simulink model "Simulate"  (R2024b)
settings: Solver=VariableStepAuto  StartTime=0.0  StopTime=Tf  FixedStep=Ti  MaxStep=Ti  RelTol=1e-6
undefined symbols (not defined in the file): CCMPC, CEMPC, DiscIntNeverNeededParam, dspblkCoreblockFVToolHelper, FOC, gcbh, IM, KF, LPF, M2C, plecs, PLL, RFT, TEB, Ti, Ts
libraries: slpidlib x4, spsdq0toAlphaBetaZeroLib x3, dspstat3 x2, spsAlphaBetaZerotoabcLib x2, embmathops x1, spsabctodq0Lib x1, spsAlphaBetaZerotodq0Lib x1, spsabctoAlphaBetaZeroLib x1
(part 1 of 2)
settings Model: Creator=Pablo  LastModifiedBy=Ingeniería Eléctrica
settings SolverCC: MinimalZcImpactIntegration=on

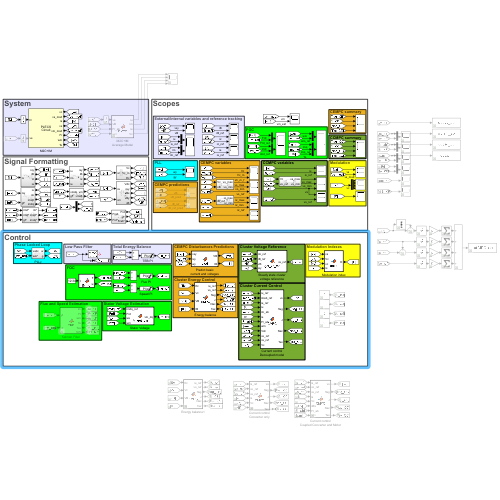
[thumbnail: Simulink's stored preview of the top-level diagram]
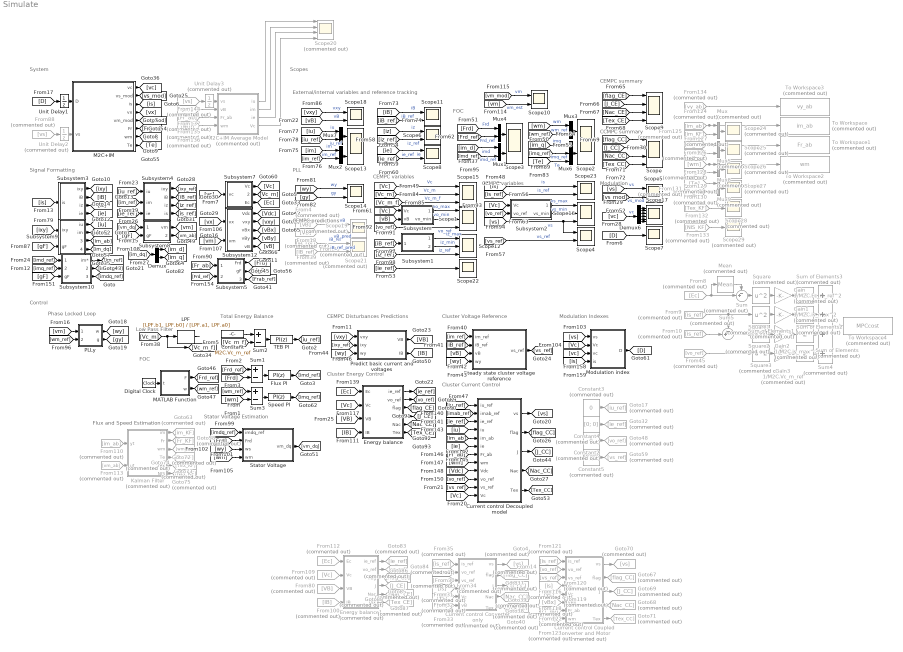
== system Simulate ==
  note: Control
  note: System
  note: Signal Formatting
  note: Scopes
  note: CEMPC predictions
  note: CEMPC variables
  note: External/internal variables and reference tracking
  note: CEMPC Disturbances Predictions
  note: FOC
  note: Cluster Energy Control
  note: Cluster Current Control
  note: Phase Locked Loop
  note: Low Pass Filter
  note: Cluster Voltage Reference
  note: PLL
  note: CEMPC summary
  note: CCMPC summary
  note: Total Energy Balance
  note: FOC
  note: CCMPC variables
  note: Modulation Indexes
  note: Flux and Speed Estimation
  note: Stator Voltage Estimation
  note: Modulation
  Constant : Constant  Value=M2C.Vc_m_ref  SampleTime=TEB.Ts
  Constant2 : Constant  Commented=on  Value=0  SampleTime=Ts
  Constant3 : Constant  Commented=on  Value=0  SampleTime=Ts
  Constant4 : Constant  Commented=on  Value=[0; 0]  SampleTime=Ts
  Constant5 : Constant  Commented=on  Value=zeros(6, 1)  SampleTime=Ts
  Current control Converter only : MATLAB Function  Commented=on  TreatAsAtomicUnit=on  SystemSampleTime=CCMPC.Ts
  Current control Coupled Converter and Motor : MATLAB Function  Commented=on  TreatAsAtomicUnit=on  SystemSampleTime=CCMPC.Ts
  Current control Decoupled model : MATLAB Function  TreatAsAtomicUnit=on  SystemSampleTime=CCMPC.Ts
  Demux : Demux  Outputs=2
  Demux6 : Demux  Outputs=M2C.m
  Digital Clock : DigitalClock  SampleTime=FOC.Ts
  Energy balance : MATLAB Function  TreatAsAtomicUnit=on  SystemSampleTime=CEMPC.Ts
  Energy balance1 : MATLAB Function  Commented=on  TreatAsAtomicUnit=on  SystemSampleTime=CEMPC.Ts
  Flux PI : slpidlib/PID Controller  Controller=PI  Form=Parallel  TimeDomain=Discrete-time  UseExternalTs=off  SampleTime=FOC.Ts  IntegratorMethod=Forward Euler  FilterMethod=Forward Euler  ControllerParametersSource=internal  P=FOC.kp_F  I=FOC.ki_F  UseKiTs=off  D=0  UseExternalDerivativeSource=off  N=100  UseFilter=on  TunerSelectOption=Transfer Function Based (PID Tuner App)  InitialConditionSource=internal  InitialConditionForIntegrator=0  InitialConditionForFilter=0  DifferentiatorICPrevScaledInput=0  ExternalReset=none  TrackingMode=off  Kt=1  LimitOutput=on  SatLimitsSource=internal  UpperSaturationLimit=FOC.u_max  LowerSaturationLimit=FOC.u_min  LinearizeAsGain=on  AntiWindupMode=back-calculation  Kb=FOC.kp_F  LimitIntegrator=off  UpperIntegratorSaturationLimit=inf  LowerIntegratorSaturationLimit=-inf  POutMin=[]  POutMax=[]  IOutMin=[]  IOutMax=[]  DOutMin=[]  DOutMax=[]  NOutMin=[]  NOutMax=[]  SumOutMin=[]  SumOutMax=[]  SaturationOutMin=[]  SaturationOutMax=[]  PParamMin=[]  PParamMax=[]  IParamMin=[]  IParamMax=[]  DParamMin=[]  DParamMax=[]  NParamMin=[]  NParamMax=[]  KbParamMin=[]  KbParamMax=[]  KtParamMin=[]  KtParamMax=[]  KbOutMin=[]  KbOutMax=[]  KtOutMin=[]  KtOutMax=[]  IntegratorOutMin=[]  IntegratorOutMax=[]  FilterOutMin=[]  FilterOutMax=[]  SumI1OutMin=[]  SumI1OutMax=[]  SumI2OutMin=[]  SumI2OutMax=[]  SumI3OutMin=[]  SumI3OutMax=[]  SumI4OutMin=[]  SumI4OutMax=[]  SumDOutMin=[]  SumDOutMax=[]  DifferentiatorOutMin=[]  DifferentiatorOutMax=[]  FilterDiffOutCoefMin=[]  FilterDiffOutCoefMax=[]  ReciprocalOutMin=[]  ReciprocalOutMax=[]  SumDenOutMin=[]  SumDenOutMax=[]  SumNumOutMin=[]  SumNumOutMax=[]  DivideOutMin=[]  DivideOutMax=[]  UdiffTsProdOutMin=[]  UdiffTsProdOutMax=[]  NTsProdOutMin=[]  NTsProdOutMax=[]  UintegralTsProdOutMin=[]  UintegralTsProdOutMax=[]  UngainTsProdOutMin=[]  UngainTsProdOutMax=[]  ClampingZeroOutDataTypeStr=Inherit: Inherit via back propagation  ClampingZeroOutMin=[]  ClampingZeroOutMax=[]  FilterDenConstantOutDataTypeStr=Inherit: Inherit via back propagation  FilterDenConstantOutMin=[]  FilterDenConstantOutMax=[]  PCopyOutDataTypeStr=Inherit: Inherit via back propagation  PCopyOutMin=[]  PCopyOutMax=[]  NCopyOutDataTypeStr=Inherit: Inherit via back propagation  NCopyOutMin=[]  NCopyOutMax=[]  IntegratorContinuousStateAttributes=''  IntegratorStateMustResolveToSignalObject=off  IntegratorRTWStateStorageClass=Auto  FilterContinuousStateAttributes=''  FilterStateMustResolveToSignalObject=off  FilterRTWStateStorageClass=Auto  ParallelPVariant=InternalParameters  IdealPVariant=Disabled  IVariant=InternalParameters  DVariant=Disabled  IntegratorVariant=Discrete  SatVariant=Enabled  AWVariant=BackCalculation  PCopyVariant=Disabled  TRVariant=Disabled  FdbkBlocksVariant=Forward  IdealPFdbkVariant=Disabled  SatFdbkVariant=Disabled  DerivativeFilterVariant=Disabled  NVariant=Disabled  NCopyVariant=Disabled_SignalSpec  FilterICVariant=Disabled  IntegratorICVariant=InternalICs  ExternalResetVariant=Disabled  TRSumVariant=Passthrough  SumFdbkVariant=Disabled  SumVariant=Sum_PI  TsampFilterVariant=InternalTs  TsampNgainVariant=Passthrough  TsampIntegralVariant=Disabled_SignalSpec  ExternalSaturationOutDataTypeStr=Inherit: Same as second input  DerivativeSourceVariant=Disabled  PreIntVariant=InternalPreInt
  From{9..10,35,121} (4 alike) : From  Commented=on  GotoTag=is_ref
  From100 : From  Commented=on  GotoTag=IB
  From109 : From  Commented=on  GotoTag=Vc
  From110 : From  Commented=on  GotoTag=im_ab
  From112 : From  Commented=on  GotoTag=Ec
  From113 : From  Commented=on  GotoTag=vm_ab
  From116 : From  Commented=on  GotoTag=vs_ref
  From118 : From  Commented=on  GotoTag=Vc
  From119 : From  Commented=on  GotoTag=vBx
  From120 : From  Commented=on  GotoTag=is
  From122 : From  Commented=on  GotoTag=Fr_ab
  From123 : From  Commented=on  GotoTag=wm
  From124 : From  Commented=on  GotoTag=im_ab
  From125 : From  Commented=on  GotoTag=im_KF
  From126 : From  Commented=on  GotoTag=Fr_ab
  From127 : From  Commented=on  GotoTag=Fr_KF
  From128 : From  Commented=on  GotoTag=wm
  From129 : From  Commented=on  GotoTag=wm_KF
  From130 : From  Commented=on  GotoTag=Te
  From131 : From  Commented=on  GotoTag=Te_KF
  From132 : From  Commented=on  GotoTag=Tex_KF
  From133 : From  Commented=on  GotoTag=NIS_KF
  From134 : From  Commented=on  GotoTag=vy_ab
  From135 : From  Commented=on  GotoTag=Fr_ab
  From136 : From  Commented=on  GotoTag=wm
  From137 : From  Commented=on  GotoTag=vB
  From14 : From  Commented=on  GotoTag=vo_ref
  From144 : From  Commented=on  GotoTag=vs
  From18 : From  Commented=on  GotoTag=VB
  From30 : From  Commented=on  GotoTag=vo_ref
  From31 : From  Commented=on  GotoTag=vs_ref
  From32 : From  Commented=on  GotoTag=Vc
  From33 : From  Commented=on  GotoTag=vB
  From34 : From  Commented=on  GotoTag=is
  From36 : From  Commented=on  GotoTag=IB_ref
  From39 : From  Commented=on  GotoTag=iB_ref
  From4 : From  Commented=on  GotoTag=vB
  From45 : From  Commented=on  GotoTag=vo_ref
  From8 : From  Commented=on  GotoTag=Ec
  From80 : From  Commented=on  GotoTag=VB
  From88 : From  Commented=on  GotoTag=vs
  Gain : Gain  Commented=on  Gain=1/M2C.Ec_m_ref^2
  Gain1 : Gain  Commented=on  Gain=1/M2C.is_max^2
  Gain2 : Gain  Commented=on  Gain=1/M2C.is_max^2
  Gain3 : Gain  Commented=on  Gain=1/M2C.Vc_m_ref
  Goto17 : Goto  Commented=on  GotoTag=iu_ref
  Goto32 : Goto  Commented=on  GotoTag=ie_ref
  Goto37 : Goto  Commented=on  GotoTag=flag_CC
  Goto38 : Goto  Commented=on  GotoTag=Nac_CC
  Goto39 : Goto  Commented=on  GotoTag=J_CC
  Goto4 : Goto  Commented=on  GotoTag=vs
  Goto40 : Goto  Commented=on  GotoTag=Tex_CC
  Goto48 : Goto  Commented=on  GotoTag=vo_ref
  Goto58 : Goto  Commented=on  GotoTag=Fr_KF
  Goto59 : Goto  Commented=on  GotoTag=vs_ref
  Goto63 : Goto  Commented=on  GotoTag=im_KF
  Goto67 : Goto  Commented=on  GotoTag=flag_CC
  Goto68 : Goto  Commented=on  GotoTag=Nac_CC
  Goto69 : Goto  Commented=on  GotoTag=J_CC
  Goto70 : Goto  Commented=on  GotoTag=vs
  Goto71 : Goto  Commented=on  GotoTag=Tex_CC
  Goto72 : Goto  Commented=on  GotoTag=wm_KF
  Goto73 : Goto  Commented=on  GotoTag=Te_KF
  Goto74 : Goto  Commented=on  GotoTag=Tex_KF
  Goto75 : Goto  Commented=on  GotoTag=NIS_KF
  Goto83 : Goto  Commented=on  GotoTag=ie_ref
  Goto84 : Goto  Commented=on  GotoTag=vo_ref
  Goto85 : Goto  Commented=on  GotoTag=flag_CE
  Goto86 : Goto  Commented=on  GotoTag=J_CE
  Goto87 : Goto  Commented=on  GotoTag=Nac_CE
  Goto88 : Goto  Commented=on  GotoTag=Tex_CE
  Kalman Filter : MATLAB Function  Commented=on  TreatAsAtomicUnit=on  SystemSampleTime=FOC.Ts
  LPF : DiscreteTransferFcn  LoadFcn=dspblkCoreblockFVToolHelper(gcbh,'load');  Numerator=[LPF.b1, LPF.b0]  Denominator=[LPF.a1, LPF.a0]  InitialStates=M2C.Vc_m_ref*9.3230807
      settings: CopyFcn=dspblkCoreblockFVToolHelper(gcbh,'copy');  DeleteFcn=dspblkCoreblockFVToolHelper(gcbh,'close');  ModelCloseFcn=dspblkCoreblockFVToolHelper(gcbh,'close');  PreSaveFcn=dspblkCoreblockFVToolHelper(gcbh,'presave');  PostSaveFcn=dspblkCoreblockFVToolHelper(gcbh,'postsave');  CloseFcn=dspblkCoreblockFVToolHelper(gcbh,'close');
  M2C+IM : Subsystem  LoadFcn=plecs('sl', 200);  InitFcn=plecs('sl', 214);  StartFcn=plecs('sl', 208);  StopFcn=plecs('sl', 209);  mask(PlecsCircuit){PLECSData=<binary blob, 34036 chars, not shown>}
      mask prompts: PLECSData "PLECS Data (Do not delete or modify!)"
      mask init:
      | % PLACE CUSTOM INITIALIZATIONS ABOVE
      | % DO NOT REMOVE
      | plecs('sl', 215);
      | % DO NOT REMOVE
      settings: CopyFcn=plecs('sl', 203);  DeleteFcn=plecs('sl', 205);  UndoDeleteFcn=plecs('sl', 206);  PreSaveFcn=plecs('sl', 211);  PostSaveFcn=plecs('sl', 201);  NameChangeFcn=plecs('sl', 210);  DestroyFcn=plecs('sl', 207);  PreCopyFcn=plecs('sl', 216);  OpenFcn=plecs('sl', 202);  ErrorFcn=plerrorfcn
      mask Help: eval('plecs(''help'', ''qthelp:///creatingacircuit.html'')')
      mask Display: disp('PLECS\nCircuit')
  M2C+IM Average Model : MATLAB Function  Commented=on  TreatAsAtomicUnit=on  SystemSampleTime=CCMPC.Ts
  MATLAB Function : MATLAB Function  TreatAsAtomicUnit=on  SystemSampleTime=FOC.Ts
  Mean : dspstat3/Mean  Commented=on  run=off  InputProcessing=Columns as channels (frame based)  reset_popup=None  directionMode=Entire input  dimension=1  roiEnable=off  roiType=Rectangles  roiPortion=Entire ROI  roiOutput=Individual statistics for each ROI  roiFlag=off  roundingMode=Floor  overflowMode=off  outputDataTypeStr=Inherit: Same as accumulator  outputMin=[]  outputMax=[]  outputLastDataTypeStr=Inherit: Same as accumulator
  Modulation index : MATLAB Function  TreatAsAtomicUnit=on  SystemSampleTime=CCMPC.Ts
  Mux : Mux  Commented=on  Inputs=[2; 2]
  Mux{1,3..4,7} (4 alike) : Mux  Inputs=2
  Mux2 : Mux  Inputs=[3; 3]
  Mux5 : Mux  Commented=on  Inputs=[2; 2]
  Mux6 : Mux  Inputs=3
  Mux8 : Mux  Commented=on  Inputs=2
  Mux9 : Mux  Commented=on  Inputs=2
  PLLy : Subsystem
  Predict basic current and voltages : MATLAB Function  TreatAsAtomicUnit=on  SystemSampleTime=CEMPC.Ts
  Scope : Scope  NumInputPorts=4
  Scope{1,12,15..16} (4 alike) : Scope  NumInputPorts=3
  Scope{2..6,8,10..11,13..14,18,23} (12 alike) : Scope  NumInputPorts=2
  Scope17 : Scope  NumInputPorts=6
  Scope19 : Scope  Commented=on  NumInputPorts=2
  Scope20 : Scope  Commented=on  NumInputPorts=4
  Scope21 : Scope  Commented=on  NumInputPorts=2
  Scope22 : Scope
  Scope{24..29} (6 alike) : Scope  Commented=on
  Scope7 : Scope
  Scope9 : Scope  NumInputPorts=4
  Speed PI : slpidlib/PID Controller  Controller=PI  Form=Parallel  TimeDomain=Discrete-time  UseExternalTs=off  SampleTime=FOC.Ts  IntegratorMethod=Forward Euler  FilterMethod=Forward Euler  ControllerParametersSource=internal  P=FOC.kp_w  I=FOC.ki_w  UseKiTs=off  D=0  UseExternalDerivativeSource=off  N=100  UseFilter=on  TunerSelectOption=Transfer Function Based (PID Tuner App)  InitialConditionSource=internal  InitialConditionForIntegrator=0  InitialConditionForFilter=0  DifferentiatorICPrevScaledInput=0  ExternalReset=none  TrackingMode=off  Kt=1  LimitOutput=on  SatLimitsSource=internal  UpperSaturationLimit=FOC.u_max  LowerSaturationLimit=FOC.u_min  LinearizeAsGain=on  AntiWindupMode=back-calculation  Kb=FOC.kp_w  LimitIntegrator=off  UpperIntegratorSaturationLimit=inf  LowerIntegratorSaturationLimit=-inf  POutMin=[]  POutMax=[]  IOutMin=[]  IOutMax=[]  DOutMin=[]  DOutMax=[]  NOutMin=[]  NOutMax=[]  SumOutMin=[]  SumOutMax=[]  SaturationOutMin=[]  SaturationOutMax=[]  PParamMin=[]  PParamMax=[]  IParamMin=[]  IParamMax=[]  DParamMin=[]  DParamMax=[]  NParamMin=[]  NParamMax=[]  KbParamMin=[]  KbParamMax=[]  KtParamMin=[]  KtParamMax=[]  KbOutMin=[]  KbOutMax=[]  KtOutMin=[]  KtOutMax=[]  IntegratorOutMin=[]  IntegratorOutMax=[]  FilterOutMin=[]  FilterOutMax=[]  SumI1OutMin=[]  SumI1OutMax=[]  SumI2OutMin=[]  SumI2OutMax=[]  SumI3OutMin=[]  SumI3OutMax=[]  SumI4OutMin=[]  SumI4OutMax=[]  SumDOutMin=[]  SumDOutMax=[]  DifferentiatorOutMin=[]  DifferentiatorOutMax=[]  FilterDiffOutCoefMin=[]  FilterDiffOutCoefMax=[]  ReciprocalOutMin=[]  ReciprocalOutMax=[]  SumDenOutMin=[]  SumDenOutMax=[]  SumNumOutMin=[]  SumNumOutMax=[]  DivideOutMin=[]  DivideOutMax=[]  UdiffTsProdOutMin=[]  UdiffTsProdOutMax=[]  NTsProdOutMin=[]  NTsProdOutMax=[]  UintegralTsProdOutMin=[]  UintegralTsProdOutMax=[]  UngainTsProdOutMin=[]  UngainTsProdOutMax=[]  ClampingZeroOutDataTypeStr=Inherit: Inherit via back propagation  ClampingZeroOutMin=[]  ClampingZeroOutMax=[]  FilterDenConstantOutDataTypeStr=Inherit: Inherit via back propagation  FilterDenConstantOutMin=[]  FilterDenConstantOutMax=[]  PCopyOutDataTypeStr=Inherit: Inherit via back propagation  PCopyOutMin=[]  PCopyOutMax=[]  NCopyOutDataTypeStr=Inherit: Inherit via back propagation  NCopyOutMin=[]  NCopyOutMax=[]  IntegratorContinuousStateAttributes=''  IntegratorStateMustResolveToSignalObject=off  IntegratorRTWStateStorageClass=Auto  FilterContinuousStateAttributes=''  FilterStateMustResolveToSignalObject=off  FilterRTWStateStorageClass=Auto  ParallelPVariant=InternalParameters  IdealPVariant=Disabled  IVariant=InternalParameters  DVariant=Disabled  IntegratorVariant=Discrete  SatVariant=Enabled  AWVariant=BackCalculation  PCopyVariant=Disabled  TRVariant=Disabled  FdbkBlocksVariant=Forward  IdealPFdbkVariant=Disabled  SatFdbkVariant=Disabled  DerivativeFilterVariant=Disabled  NVariant=Disabled  NCopyVariant=Disabled_SignalSpec  FilterICVariant=Disabled  IntegratorICVariant=InternalICs  ExternalResetVariant=Disabled  TRSumVariant=Passthrough  SumFdbkVariant=Disabled  SumVariant=Sum_PI  TsampFilterVariant=InternalTs  TsampNgainVariant=Passthrough  TsampIntegralVariant=Disabled_SignalSpec  ExternalSaturationOutDataTypeStr=Inherit: Same as second input  DerivativeSourceVariant=Disabled  PreIntVariant=InternalPreInt
  Square{,1..3} (4 alike) : Math  Commented=on  Operator=square
  Stator Voltage : MATLAB Function  TreatAsAtomicUnit=on  SystemSampleTime=CCMPC.Ts
  Steady state cluster voltage reference : MATLAB Function  TreatAsAtomicUnit=on  SystemSampleTime=CCMPC.Ts
  Subsystem : Subsystem
  Subsystem1 : Subsystem
  Subsystem10 : Subsystem
  Subsystem12 : Subsystem
  Subsystem2 : Subsystem
  Subsystem3 : Subsystem
  Subsystem4 : Subsystem
  Subsystem5 : Subsystem
  Subsystem7 : Subsystem
  Subsystem8 : Subsystem
  Subsystem9 : Subsystem
  Sum : Sum  Commented=on  Inputs=-+|
  Sum of Elements{,1..3} (4 alike) : Sum  Commented=on  Inputs=+
  Sum1 : Sum  Inputs=+-
  Sum2 : Sum  Inputs=+-
  Sum3 : Sum  Inputs=+-
  Sum4 : Sum  Commented=on  Inputs=++++
  Sum5 : Sum  Commented=on  Inputs=-+|
  TEB PI : slpidlib/PID Controller  Controller=PI  Form=Parallel  TimeDomain=Discrete-time  UseExternalTs=off  SampleTime=TEB.Ts  IntegratorMethod=Forward Euler  FilterMethod=Forward Euler  ControllerParametersSource=internal  P=TEB.kp  I=TEB.ki  UseKiTs=off  D=0  UseExternalDerivativeSource=off  N=100  UseFilter=on  TunerSelectOption=Transfer Function Based (PID Tuner App)  InitialConditionSource=internal  InitialConditionForIntegrator=0  InitialConditionForFilter=0  DifferentiatorICPrevScaledInput=0  ExternalReset=none  TrackingMode=off  Kt=1  LimitOutput=on  SatLimitsSource=internal  UpperSaturationLimit=TEB.u_max  LowerSaturationLimit=TEB.u_min  LinearizeAsGain=on  AntiWindupMode=clamping  Kb=1  LimitIntegrator=off  UpperIntegratorSaturationLimit=inf  LowerIntegratorSaturationLimit=-inf  POutMin=[]  POutMax=[]  IOutMin=[]  IOutMax=[]  DOutMin=[]  DOutMax=[]  NOutMin=[]  NOutMax=[]  SumOutMin=[]  SumOutMax=[]  SaturationOutMin=[]  SaturationOutMax=[]  PParamMin=[]  PParamMax=[]  IParamMin=[]  IParamMax=[]  DParamMin=[]  DParamMax=[]  NParamMin=[]  NParamMax=[]  KbParamMin=[]  KbParamMax=[]  KtParamMin=[]  KtParamMax=[]  KbOutMin=[]  KbOutMax=[]  KtOutMin=[]  KtOutMax=[]  IntegratorOutMin=[]  IntegratorOutMax=[]  FilterOutMin=[]  FilterOutMax=[]  SumI1OutMin=[]  SumI1OutMax=[]  SumI2OutMin=[]  SumI2OutMax=[]  SumI3OutMin=[]  SumI3OutMax=[]  SumI4OutMin=[]  SumI4OutMax=[]  SumDOutMin=[]  SumDOutMax=[]  DifferentiatorOutMin=[]  DifferentiatorOutMax=[]  FilterDiffOutCoefMin=[]  FilterDiffOutCoefMax=[]  ReciprocalOutMin=[]  ReciprocalOutMax=[]  SumDenOutMin=[]  SumDenOutMax=[]  SumNumOutMin=[]  SumNumOutMax=[]  DivideOutMin=[]  DivideOutMax=[]  UdiffTsProdOutMin=[]  UdiffTsProdOutMax=[]  NTsProdOutMin=[]  NTsProdOutMax=[]  UintegralTsProdOutMin=[]  UintegralTsProdOutMax=[]  UngainTsProdOutMin=[]  UngainTsProdOutMax=[]  ClampingZeroOutDataTypeStr=Inherit: Inherit via back propagation  ClampingZeroOutMin=[]  ClampingZeroOutMax=[]  FilterDenConstantOutDataTypeStr=Inherit: Inherit via back propagation  FilterDenConstantOutMin=[]  FilterDenConstantOutMax=[]  PCopyOutDataTypeStr=Inherit: Inherit via back propagation  PCopyOutMin=[]  PCopyOutMax=[]  NCopyOutDataTypeStr=Inherit: Inherit via back propagation  NCopyOutMin=[]  NCopyOutMax=[]  IntegratorContinuousStateAttributes=''  IntegratorStateMustResolveToSignalObject=off  IntegratorRTWStateStorageClass=Auto  FilterContinuousStateAttributes=''  FilterStateMustResolveToSignalObject=off  FilterRTWStateStorageClass=Auto  ParallelPVariant=InternalParameters  IdealPVariant=Disabled  IVariant=InternalParameters  DVariant=Disabled  IntegratorVariant=Discrete  SatVariant=Enabled  AWVariant=DiscClampingParallel  PCopyVariant=Disabled  TRVariant=Disabled  FdbkBlocksVariant=Forward  IdealPFdbkVariant=Disabled  SatFdbkVariant=Disabled  DerivativeFilterVariant=Disabled  NVariant=Disabled  NCopyVariant=Disabled_SignalSpec  FilterICVariant=Disabled  IntegratorICVariant=InternalICs  ExternalResetVariant=Disabled  TRSumVariant=Passthrough  SumFdbkVariant=Disabled  SumVariant=Sum_PI  TsampFilterVariant=InternalTs  TsampNgainVariant=Passthrough  TsampIntegralVariant=Disabled_SignalSpec  ExternalSaturationOutDataTypeStr=Inherit: Same as second input  DerivativeSourceVariant=Disabled  PreIntVariant=InternalPreInt
  To Workspace : ToWorkspace  Commented=on  VariableName=im_ab  SaveFormat=Timeseries  SampleTime=FOC.Ts
  To Workspace1 : ToWorkspace  Commented=on  VariableName=Fr_ab  SaveFormat=Timeseries  SampleTime=FOC.Ts
  To Workspace2 : ToWorkspace  Commented=on  VariableName=wm  SaveFormat=Timeseries  SampleTime=FOC.Ts
  To Workspace3 : ToWorkspace  Commented=on  VariableName=vy_ab  SaveFormat=Timeseries  SampleTime=FOC.Ts
  To Workspace4 : ToWorkspace  Commented=on  VariableName=MPCcost  SaveFormat=Timeseries  SampleTime=Ts
  Unit Delay1 : UnitDelay  InitialCondition=zeros(24, 1)  SampleTime=Ti  HasFrameUpgradeWarning=on
  Unit Delay2 : UnitDelay  Commented=on  InitialCondition=zeros(6, 1)  SampleTime=Ti  HasFrameUpgradeWarning=on
  Unit Delay3 : UnitDelay  Commented=on  InitialCondition=zeros(6, 1)  SampleTime=Ti  HasFrameUpgradeWarning=on
  wires:
  From14/1 -> Current control Coupled Converter and Motor/2(vo_ref)
  From120/1 -> Current control Coupled Converter and Motor/4(is)
  From119/1 -> Current control Coupled Converter and Motor/6(vBx)
  Current control Coupled Converter and Motor/3(J) -> Goto69/1
  Current control Coupled Converter and Motor/2(flag) -> Goto67/1
  From121/1 -> Current control Coupled Converter and Motor/1(is_ref)
  Current control Coupled Converter and Motor/1(vs) -> Goto70/1
  Current control Coupled Converter and Motor/5(Tex) -> Goto71/1
  Current control Coupled Converter and Motor/4(Nac) -> Goto68/1
  From118/1 -> Current control Coupled Converter and Motor/5(Vc)
  From116/1 -> Current control Coupled Converter and Motor/3(vs_ref)
  From122/1 -> Current control Coupled Converter and Motor/7(Fr_ab)
  From123/1 -> Current control Coupled Converter and Motor/8(wm)
  From125/1 -> Mux/2
  From132/1 -> Scope28/1
  From126/1 -> To Workspace1/1, Mux5/1
  From131/1 -> Mux9/2
  From129/1 -> Mux8/2
  From130/1 -> Mux9/1
  From128/1 -> To Workspace2/1, Mux8/1
  From127/1 -> Mux5/2
  Mux/1 -> Scope24/1
  Mux5/1 -> Scope25/1
  Mux8/1 -> Scope26/1
  Mux9/1 -> Scope27/1
  From133/1 -> Scope29/1
  From124/1 -> To Workspace/1, Mux/1
  From134/1 -> To Workspace3/1
  From8/1 -> Sum/2, Mean/1
  Sum/1 -> Square/1
  From9/1 -> Sum5/1, Square1/1
  Square1/1 -> Gain1/1
  Square/1 -> Gain/1
  Square2/1 -> Gain2/1
  Mean/1 -> Sum/1
  From45/1 -> Square3/1
  Sum4/1 -> To Workspace4/1
  Sum5/1 -> Square2/1
  From10/1 -> Sum5/2
  Square3/1 -> Gain3/1
  Gain/1 -> Sum of Elements3/1
  Gain1/1 -> Sum of Elements2/1
  Gain2/1 -> Sum of Elements1/1
  Gain3/1 -> Sum of Elements/1
  Sum of Elements/1 -> Sum4/4
  Sum of Elements1/1 -> Sum4/3
  Sum of Elements2/1 -> Sum4/2
  Sum of Elements3/1 -> Sum4/1
  [iu] -> Current control Decoupled model/4(iu)
  [ie_ref] -> Current control Decoupled model/3(ie_ref)
  [imab_ref] -> Current control Decoupled model/2(imab_ref)
  [iu_ref] -> Current control Decoupled model/1(iu_ref)
  [im_ab] -> Current control Decoupled model/5(im_ab)
  [ie] -> Current control Decoupled model/6(ie)
  [Fr_ab] -> Current control Decoupled model/7(Fr_ab)
  [wm] -> Current control Decoupled model/8(wm)
  [Vdc] -> Current control Decoupled model/9(Vdc)
  [vo_ref] -> Current control Decoupled model/10(vo_ref)
  Current control Decoupled model/1(vs) -> [vs]
  [Vc] -> Current control Decoupled model/12(Vc)
  Current control Decoupled model/2(flag) -> [flag_CC]
  Current control Decoupled model/3(J) -> [J_CC]
  Current control Decoupled model/4(Nac) -> [Nac_CC]
  Current control Decoupled model/5(Tex) -> [Tex_CC]
  [vs_ref] -> Current control Decoupled model/11(vs_ref)
  Energy balance1/3(flag) -> Goto85/1
  Energy balance1/6(Tex) -> Goto88/1
  Energy balance1/4(J) -> Goto86/1
  Energy balance1/1(ie_ref) -> Goto83/1
  From80/1 -> Energy balance1/3(VB)
  From109/1 -> Energy balance1/2(Vc)
  Energy balance1/5(Nac) -> Goto87/1
  From112/1 -> Energy balance1/1(Ec)
  Energy balance1/2(vo_ref) -> Goto84/1
  From100/1 -> Energy balance1/4(IB)
  From31/1 -> Current control Converter only/3(vs_ref)
  From34/1 -> Current control Converter only/4(is)
  Current control Converter only/4(Nac) -> Goto38/1
  From33/1 -> Current control Converter only/6(vB)
  Current control Converter only/3(J) -> Goto39/1
  From32/1 -> Current control Converter only/5(Vc)
  From30/1 -> Current control Converter only/2(vo_ref)
  From35/1 -> Current control Converter only/1(is_ref)
  Current control Converter only/2(flag) -> Goto37/1
  Current control Converter only/5(Tex) -> Goto40/1
  Current control Converter only/1(vs) -> Goto4/1
  [im_dq] -> Demux/1
  Demux/2 -> [im_q]
  [gF] -> Subsystem10/3(gF)
  [imq_ref] -> Subsystem10/2(imq*)
  Demux/1 -> [im_d]
  Subsystem10/1(im*) -> [im_ref]
  PLLy/1(w) -> [wy]
  Subsystem/2(vo_min) -> Scope1/2  "vo_min"
  [vs_mod] -> Scope5/2  "vs_mod"
  [wm_ref] -> PLLy/2(wm*)
  [ixy_ref] -> Predict basic current and voltages/2(ixy)
  Subsystem4/3(iz) -> [iz_ref]
  MATLAB Function/2(w) -> [wm_ref]
  From113/1 -> Kalman Filter/2(ut)
  [Nac_CC] -> Scope/3
  [J_CC] -> Scope/2
  Constant4/1 -> Goto32/1
  Kalman Filter/5(Tex) -> Goto74/1
  [Frd_ref] -> Mux4/2  "Frd_ref"
  Kalman Filter/6(NIS) -> Goto75/1
  [vs] -> Modulation index/1(vs)
  [wm_ref] -> Sum3/1
  Subsystem3/4(ie) -> [ie]
  From4/1 -> Scope19/1  "vB"
  [Vc] -> Modulation index/2(Vc)
  [Vc_m_f] -> Scope15/3  "Vc_m_f"
  [J_CE] -> Scope9/2
  [Tex_CE] -> Scope9/4
  M2C+IM/4(vx) -> [vx]
  Unit Delay3/1 -> M2C+IM Average Model/1(vs)
  [vx] -> Subsystem12/1(vx)
  [D] -> Scope7/1
  Subsystem7/1(Vc) -> [Vc]
  Subsystem2/1(vs_max) -> Scope16/1  "vs_max"
  [vB] -> Scope18/2  "vB"
  Subsystem3/1(ixy) -> [ixy]
  [im] -> Mux2/1  "im"
  [iu] -> Mux7/1  "iu"
  [wy] -> Stator Voltage/3(ws)
  Subsystem12/2(vxy) -> [vxy]
  [imq_ref] -> Mux6/2  "imq_ref"
  [iB_ref] -> Steady state cluster voltage reference/2(iB_ref)
  [vB] -> Subsystem/2(vB)
  Subsystem8/2(vmαβ) -> [vm_ab]
  [Vc] -> Subsystem/1(Vc)
  M2C+IM/2(vs_mod) -> [vs_mod]
  Sum2/1 -> TEB PI/1
  [vm] -> Scope10/2  "vm_est"
  Subsystem5/3(Frab*) -> [Frab_ref]
  [im_ref] -> Mux2/2  "im_ref"
  [vo_ref] -> Scope1/3  "vo_ref"
  [ie_ref] -> Scope22/1
  [wy] -> Predict basic current and voltages/3(wy)
  Subsystem9/1(iu) -> [iu]
  Subsystem1/2(iz_min) -> Scope12/2  "iz_min"
  [Fr_ab] -> Subsystem5/1(Frab)
  Mux3/1 -> Scope2/1
  Subsystem12/3(vBx) -> [vBx]
  Subsystem5/1(Frd) -> [Frd]
  Subsystem/1(vo_max) -> Scope1/1  "vo_max"
  Constant2/1 -> Goto48/1
  M2C+IM/5(vm_mod) -> [vm_mod]
  [im_ref] -> Subsystem4/2(im)
  [iu_ref] -> Mux7/2  "iu_ref"
  Sum3/1 -> Speed PI/1
  [gF] -> Subsystem8/2(gF)
  [wm] -> Sum3/2
  [vs_ref] -> Scope4/2  "vs_ref"
  [ie_ref] -> Subsystem4/3(ie)
  Mux6/1 -> Scope2/2
  Flux PI/1 -> [imd_ref]
  [imd_ref] -> Mux1/2  "imd_ref"
  Subsystem12/1(Vdc) -> [Vdc]
  Demux6/1 -> Scope17/1
  [vxy] -> Predict basic current and voltages/1(vxy)
  Demux6/3 -> Scope17/3
  Demux6/5 -> Scope17/5
  [vs] -> Scope4/1, Scope16/3  "vs"
  From39/1 -> Scope21/1  "iB_ref"
  MATLAB Function/1(F) -> [Frd_ref]
  Subsystem7/2(Vc_m) -> [Vc_m]
  Mux2/1 -> Scope13/2
  [vm_dq] -> Subsystem8/1(vmdq)
  Subsystem5/2(gF) -> [gF]
  [gy] -> Scope14/2  "gy"
  Subsystem10/2(imαβ*) -> [imab_ref]
  [vm] -> PLLy/1(vabc)
  Subsystem9/3(imαβ) -> [im_ab]
  PLLy/2(g) -> [gy]
  Subsystem10/3(imdq*) -> [imdq_ref]
  Modulation index/1(D) -> [D]
  Subsystem4/2(iB) -> [iB_ref]
  Predict basic current and voltages/2(IB) -> [IB]
  [vB] -> Steady state cluster voltage reference/3(vB)
  Subsystem9/2(im) -> [im]
  [wy] -> Scope14/1  "wy"
  Subsystem2/2(vs_min) -> Scope16/2  "vs_min"
  Kalman Filter/4(Te) -> Goto73/1
  From88/1 -> Unit Delay2/1
  [iu_ref] -> Subsystem4/1(iu)
  TEB PI/1 -> [iu_ref]
  [Vc_m] -> Scope15/2  "Vc_m"
  [iz] -> Scope6/1  "iz"
  [ie_ref] -> Scope8/2  "ie_ref"
  Kalman Filter/3(wm) -> Goto72/1
  Kalman Filter/2(Fr) -> Goto58/1
  [flag_CC] -> Scope/1
  Constant3/1 -> Goto17/1
  [wm] -> Stator Voltage/4(wm)
  Mux1/1 -> Scope3/2
  [im_q] -> Mux6/1  "imq"
  Stator Voltage/1(vm_dq) -> [vm_dq]
  [iB_ref] -> Scope11/2  "iB_ref"
  M2C+IM/8(Te) -> [Te]
  Steady state cluster voltage reference/1(vs_ref) -> [vs_ref]
  [D] -> Unit Delay1/1
  From36/1 -> Scope21/2  "iB_ref_pred"
  [iz_ref] -> Scope12/3  "iz_ref"
  Kalman Filter/1(im) -> Goto63/1
  [Frd_ref] -> Sum1/1
  [Vc] -> Subsystem2/1(Vc)
  Subsystem7/3(Ec) -> [Ec]
  Subsystem8/1(vm) -> [vm]
  [vc] -> Modulation index/3(vc)
  Sum1/1 -> Flux PI/1
  [im_ref] -> Steady state cluster voltage reference/1(im_ref)
  Subsystem3/2(iB) -> [iB]
  Demux6/4 -> Scope17/4
  [wm_ref] -> Mux3/2  "wm_ref"
  Unit Delay2/1 -> M2C+IM/2(vs)
  [vm] -> Subsystem12/2(vm)
  [Frd] -> Sum1/2
  [Frd] -> Mux4/1  "Frd"
  [iB] -> Scope11/1  "iB"
  Predict basic current and voltages/1(VB) -> [VB]
  [is] -> Subsystem3/1(is)
  Mux7/1 -> Scope13/1
  [iB_ref] -> Subsystem1/1(iB_ref)
  [wm] -> Mux3/1  "wm"
  [imdq_ref] -> Stator Voltage/1(imdq_ref)
  [imd_ref] -> Subsystem10/1(imd*)
  M2C+IM/6(Fr) -> [Fr_ab]
  Constant/1 -> Sum2/1
  [flag_CE] -> Scope9/1
  Subsystem4/4(is) -> [is_ref]
  [vc] -> Demux6/1  "vc"
  [is_ref] -> Scope23/2  "is_ref"
  Constant5/1 -> Goto59/1
  Subsystem4/1(ixy) -> [ixy_ref]
  [wy] -> Steady state cluster voltage reference/4(wy)
  [iz_ref] -> Scope6/2  "iz_ref"
  Mux4/1 -> Scope3/1
  [Frd_ref] -> Subsystem5/2(Frd*)
  Demux6/2 -> Scope17/2
  LPF/1 -> ?
  M2C+IM/7(wm) -> [wm]
  Subsystem12/4(vBy) -> [vBy]
  [Frd] -> Stator Voltage/2(Frd)
  From18/1 -> Scope19/2  "vB_pred"
  Subsystem9/4(imdq) -> [im_dq]
  M2C+IM/3(is) -> [is]
  [im_d] -> Mux1/1  "imd"
  From110/1 -> Kalman Filter/1(yt)
  [vs] -> Scope5/1  "vs"
  [Nac_CE] -> Scope9/3
  [is] -> Scope23/1  "is"
  Subsystem3/3(iz) -> [iz]
  From144/1 -> Unit Delay3/1
  [Tex_CC] -> Scope/4
  [vc] -> Subsystem7/1(vc)
  [vxy] -> Scope18/1  "vxy"
  [Vc_m_f] -> Sum2/2
  Digital Clock/1 -> MATLAB Function/1(t)
  Speed PI/1 -> [imq_ref]
  Subsystem12/5(vB) -> [vB]
  [vm_mod] -> Scope10/1  "vm"
  [ie] -> Scope8/1  "ie"
  [gF] -> Subsystem9/2(gF)
  M2C+IM/1(vc) -> [vc]
  [vo_ref] -> Subsystem2/2(vo_ref)
  [Te] -> Mux6/3  "Te"
  Unit Delay1/1 -> M2C+IM/1(D)
  Subsystem1/1(iz_max) -> Scope12/1  "iz_max"
  Demux6/6 -> Scope17/6
  [Vc] -> Scope15/1  "Vc"
  [is] -> Modulation index/4(is)
  [ixy] -> Subsystem9/1(ixy)
  Energy balance/2(vo_ref) -> [vo_ref]
  Energy balance/5(Nac) -> [Nac_CE]
  [Vc] -> Energy balance/2(Vc)
  [Ec] -> Energy balance/1(Ec)
  Energy balance/3(flag) -> [flag_CE]
  [VB] -> Energy balance/3(VB)
  Energy balance/1(ie_ref) -> [ie_ref]
  Energy balance/4(J) -> [J_CE]
  Energy balance/6(Tex) -> [Tex_CE]
  [IB] -> Energy balance/4(IB)
  From135/1 -> M2C+IM Average Model/3(Fr_ab)
  From136/1 -> M2C+IM Average Model/4(wm)
  M2C+IM Average Model/1(iu) -> Scope20/1
  M2C+IM Average Model/2(im) -> Scope20/2
  M2C+IM Average Model/3(ie) -> Scope20/3
  M2C+IM Average Model/4(Vc) -> Scope20/4
  From137/1 -> M2C+IM Average Model/2(vB)
  [Vc_m] -> [Vc_m_f], LPF/1

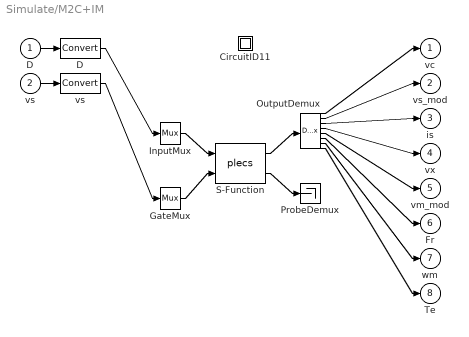
== system Simulate/M2C+IM ==
  D : Inport  PortDimensions=24
  vs : Inport  Port=2  PortDimensions=6
  " CircuitID11 " : Subsystem
  " D " : DataTypeConversion
  " GateMux " : Mux  Inputs=[ 6 ]
  " InputMux " : Mux  Inputs=[ 24 ]
  " OutputDemux " : Demux  Outputs=[ 24 6 6 2 3 2 1 1 ]
  " ProbeDemux " : Terminator
  " S-Function " : S-Function  FunctionName=plecs  SFunctionDeploymentMode=off  EnableBusSupport=off
  " vs " : DataTypeConversion
  vc : Outport  PortDimensions=24
  vs_mod : Outport  Port=2  PortDimensions=6
  is : Outport  Port=3  PortDimensions=6
  vx : Outport  Port=4  PortDimensions=2
  vm_mod : Outport  Port=5  PortDimensions=3
  Fr : Outport  Port=6  PortDimensions=2
  wm : Outport  Port=7  PortDimensions=1
  Te : Outport  Port=8  PortDimensions=1
  wires:
  " InputMux "/1 -> " S-Function "/1
  " GateMux "/1 -> " S-Function "/2
  " S-Function "/1 -> " OutputDemux "/1
  " S-Function "/2 -> " ProbeDemux "/1
  D/1 -> " D "/1
  " D "/1 -> " InputMux "/1
  vs/1 -> " vs "/1
  " vs "/1 -> " GateMux "/1
  " OutputDemux "/1 -> vc/1
  " OutputDemux "/2 -> vs_mod/1
  " OutputDemux "/3 -> is/1
  " OutputDemux "/4 -> vx/1
  " OutputDemux "/5 -> vm_mod/1
  " OutputDemux "/6 -> Fr/1
  " OutputDemux "/7 -> wm/1
  " OutputDemux "/8 -> Te/1

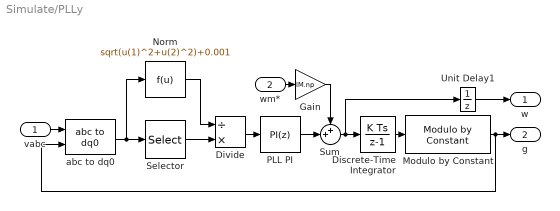
== system Simulate/PLLy ==
  vabc : Inport
  wm* : Inport  Port=2
  Discrete-Time Integrator : DiscreteIntegrator  SampleTime=PLL.Ts  ICPrevOutput=DiscIntNeverNeededParam  ICPrevScaledInput=DiscIntNeverNeededParam
  Divide : Product  Inputs=/*
  Gain : Gain  Gain=IM.np
  Modulo by Constant : embmathops/Modulo by Constant  Denominator=2*pi  SimulateUsing=Code generation
  Norm : Fcn  Expr=sqrt(u(1)^2+u(2)^2)+0.001
  PLL PI : slpidlib/PID Controller  Controller=PI  Form=Parallel  TimeDomain=Discrete-time  UseExternalTs=off  SampleTime=PLL.Ts  IntegratorMethod=Forward Euler  FilterMethod=Forward Euler  ControllerParametersSource=internal  P=PLL.kp  I=PLL.ki  UseKiTs=off  D=0  UseExternalDerivativeSource=off  N=100  UseFilter=on  TunerSelectOption=Transfer Function Based (PID Tuner App)  InitialConditionSource=internal  InitialConditionForIntegrator=0  InitialConditionForFilter=0  DifferentiatorICPrevScaledInput=0  ExternalReset=none  TrackingMode=off  Kt=1  LimitOutput=off  SatLimitsSource=internal  UpperSaturationLimit=inf  LowerSaturationLimit=-inf  LinearizeAsGain=on  AntiWindupMode=none  Kb=1  LimitIntegrator=off  UpperIntegratorSaturationLimit=inf  LowerIntegratorSaturationLimit=-inf  POutMin=[]  POutMax=[]  IOutMin=[]  IOutMax=[]  DOutMin=[]  DOutMax=[]  NOutMin=[]  NOutMax=[]  SumOutMin=[]  SumOutMax=[]  SaturationOutMin=[]  SaturationOutMax=[]  PParamMin=[]  PParamMax=[]  IParamMin=[]  IParamMax=[]  DParamMin=[]  DParamMax=[]  NParamMin=[]  NParamMax=[]  KbParamMin=[]  KbParamMax=[]  KtParamMin=[]  KtParamMax=[]  KbOutMin=[]  KbOutMax=[]  KtOutMin=[]  KtOutMax=[]  IntegratorOutMin=[]  IntegratorOutMax=[]  FilterOutMin=[]  FilterOutMax=[]  SumI1OutMin=[]  SumI1OutMax=[]  SumI2OutMin=[]  SumI2OutMax=[]  SumI3OutMin=[]  SumI3OutMax=[]  SumI4OutMin=[]  SumI4OutMax=[]  SumDOutMin=[]  SumDOutMax=[]  DifferentiatorOutMin=[]  DifferentiatorOutMax=[]  FilterDiffOutCoefMin=[]  FilterDiffOutCoefMax=[]  ReciprocalOutMin=[]  ReciprocalOutMax=[]  SumDenOutMin=[]  SumDenOutMax=[]  SumNumOutMin=[]  SumNumOutMax=[]  DivideOutMin=[]  DivideOutMax=[]  UdiffTsProdOutMin=[]  UdiffTsProdOutMax=[]  NTsProdOutMin=[]  NTsProdOutMax=[]  UintegralTsProdOutMin=[]  UintegralTsProdOutMax=[]  UngainTsProdOutMin=[]  UngainTsProdOutMax=[]  ClampingZeroOutDataTypeStr=Inherit: Inherit via back propagation  ClampingZeroOutMin=[]  ClampingZeroOutMax=[]  FilterDenConstantOutDataTypeStr=Inherit: Inherit via back propagation  FilterDenConstantOutMin=[]  FilterDenConstantOutMax=[]  PCopyOutDataTypeStr=Inherit: Inherit via back propagation  PCopyOutMin=[]  PCopyOutMax=[]  NCopyOutDataTypeStr=Inherit: Inherit via back propagation  NCopyOutMin=[]  NCopyOutMax=[]  IntegratorContinuousStateAttributes=''  IntegratorStateMustResolveToSignalObject=off  IntegratorRTWStateStorageClass=Auto  FilterContinuousStateAttributes=''  FilterStateMustResolveToSignalObject=off  FilterRTWStateStorageClass=Auto  ParallelPVariant=InternalParameters  IdealPVariant=Disabled  IVariant=InternalParameters  DVariant=Disabled  IntegratorVariant=Discrete  SatVariant=Disabled  AWVariant=Passthrough  PCopyVariant=Disabled  TRVariant=Disabled  FdbkBlocksVariant=Forward  IdealPFdbkVariant=Disabled  SatFdbkVariant=Disabled  DerivativeFilterVariant=Disabled  NVariant=Disabled  NCopyVariant=Disabled_SignalSpec  FilterICVariant=Disabled  IntegratorICVariant=InternalICs  ExternalResetVariant=Disabled  TRSumVariant=Passthrough  SumFdbkVariant=Disabled  SumVariant=Sum_PI  TsampFilterVariant=InternalTs  TsampNgainVariant=Passthrough  TsampIntegralVariant=Disabled_SignalSpec  ExternalSaturationOutDataTypeStr=Inherit: Same as second input  DerivativeSourceVariant=Disabled  PreIntVariant=InternalPreInt
  Selector : Selector  InputPortWidth=3  IndexOptions=Index vector (dialog)  Indices=[2]  OutputSizes=1
  Sum : Sum  Inputs=++|
  Unit Delay1 : UnitDelay  SampleTime=Ti  HasFrameUpgradeWarning=on
  abc to dq0 : spsabctodq0Lib/abc to dq0  Alignment=Aligned with phase A axis
  w : Outport
  g : Outport  Port=2
  wires:
  Divide/1 -> PLL PI/1
  Discrete-Time Integrator/1 -> Modulo by Constant/1
  Selector/1 -> Divide/2
  Modulo by Constant/1 -> abc to dq0/2, g/1
  PLL PI/1 -> Sum/2
  Sum/1 -> Unit Delay1/1, Discrete-Time Integrator/1
  wm*/1 -> Gain/1
  Gain/1 -> Sum/1
  vabc/1 -> abc to dq0/1
  Unit Delay1/1 -> w/1
  abc to dq0/1 -> Norm/1, Selector/1
  Norm/1 -> Divide/1

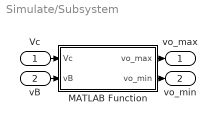
== system Simulate/Subsystem ==
  Vc : Inport
  vB : Inport  Port=2
  MATLAB Function : MATLAB Function  TreatAsAtomicUnit=on
  vo_max : Outport
  vo_min : Outport  Port=2
  wires:
  MATLAB Function/1(vo_max) -> vo_max/1
  MATLAB Function/2(vo_min) -> vo_min/1
  Vc/1 -> MATLAB Function/1(Vc)
  vB/1 -> MATLAB Function/2(vB)

== system Simulate/Subsystem1 ==
  iB_ref : Inport
  MATLAB Function : MATLAB Function  TreatAsAtomicUnit=on  SystemSampleTime=Ts
  iz_max : Outport
  iz_min : Outport  Port=2
  wires:
  MATLAB Function/1(iz_max) -> iz_max/1
  MATLAB Function/2(iz_min) -> iz_min/1
  iB_ref/1 -> MATLAB Function/1(iB_ref)

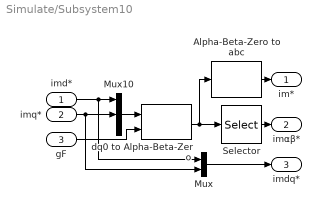
== system Simulate/Subsystem10 ==
  imd* : Inport
  imq* : Inport  Port=2
  gF : Inport  Port=3
  Alpha-Beta-Zero to abc : spsAlphaBetaZerotoabcLib/Alpha-Beta-Zero to abc
  Mux : Mux  Inputs=2
  Mux10 : Mux  Inputs=3
  Selector : Selector  InputPortWidth=3  IndexOptions=Index vector (dialog)  Indices=[1 2]  OutputSizes=1
  dq0 to Alpha-Beta-Zero : spsdq0toAlphaBetaZeroLib/dq0 to Alpha-Beta-Zero  Alignment=Aligned with phase A axis
  im* : Outport
  imαβ* : Outport  Port=2
  imdq* : Outport  Port=3
  wires:
  dq0 to Alpha-Beta-Zero/1 -> Alpha-Beta-Zero to abc/1, Selector/1
  gF/1 -> dq0 to Alpha-Beta-Zero/2
  Mux10/1 -> dq0 to Alpha-Beta-Zero/1
  Selector/1 -> imαβ*/1
  imd*/1 -> Mux/1, Mux10/1
  Alpha-Beta-Zero to abc/1 -> im*/1
  imq*/1 -> Mux10/2, Mux/2
  Mux/1 -> imdq*/1

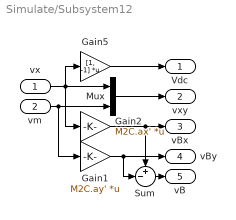
== system Simulate/Subsystem12 ==
  vx : Inport
  vm : Inport  Port=2
  Gain1 : Gain  Gain=M2C.ay'  Multiplication=Matrix(K*u)
  Gain2 : Gain  Gain=M2C.ax'  Multiplication=Matrix(K*u)
  Gain5 : Gain  Gain=[1, -1]  Multiplication=Matrix(K*u)
  Mux : Mux  Inputs=[2; 3]
  Sum : Sum  Inputs=+-|
  Vdc : Outport
  vxy : Outport  Port=2
  vBx : Outport  Port=3
  vBy : Outport  Port=4
  vB : Outport  Port=5
  wires:
  Mux/1 -> vxy/1
  vx/1 -> Gain5/1, Gain2/1, Mux/1
  Gain2/1 -> Sum/1, vBx/1
  Gain1/1 -> Sum/2, vBy/1
  Sum/1 -> vB/1
  vm/1 -> Mux/2, Gain1/1
  Gain5/1 -> Vdc/1

== system Simulate/Subsystem2 ==
  Vc : Inport
  vo_ref : Inport  Port=2
  MATLAB Function : MATLAB Function  TreatAsAtomicUnit=on  SystemSampleTime=Ts
  vs_max : Outport
  vs_min : Outport  Port=2
  wires:
  MATLAB Function/2(vs_min) -> vs_min/1
  Vc/1 -> MATLAB Function/1(Vc)
  MATLAB Function/1(vs_max) -> vs_max/1
  vo_ref/1 -> MATLAB Function/2(vo_ref)

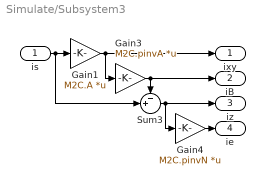
== system Simulate/Subsystem3 ==
  is : Inport
  Gain1 : Gain  Gain=M2C.A  Multiplication=Matrix(K*u)
  Gain3 : Gain  Gain=M2C.pinvA  Multiplication=Matrix(K*u)
  Gain4 : Gain  Gain=M2C.pinvN  Multiplication=Matrix(K*u)
  Sum3 : Sum  Inputs=-+|
  ixy : Outport
  iB : Outport  Port=2
  iz : Outport  Port=3
  ie : Outport  Port=4
  wires:
  Gain3/1 -> iB/1, Sum3/1
  is/1 -> Sum3/2, Gain1/1
  Gain1/1 -> ixy/1, Gain3/1
  Sum3/1 -> iz/1, Gain4/1
  Gain4/1 -> ie/1

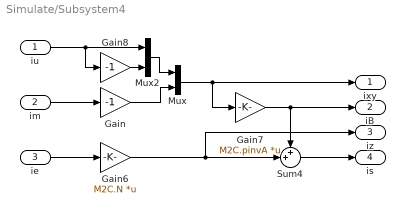
== system Simulate/Subsystem4 ==
  iu : Inport
  im : Inport  Port=2
  ie : Inport  Port=3
  Gain : Gain  Gain=-1
  Gain6 : Gain  Gain=M2C.N  Multiplication=Matrix(K*u)
  Gain7 : Gain  Gain=M2C.pinvA  Multiplication=Matrix(K*u)
  Gain8 : Gain  Gain=-1
  Mux : Mux  Inputs=[M2C.p; M2C.q]
  Mux2 : Mux  Inputs=2
  Sum4 : Sum  Inputs=++|
  ixy : Outport
  iB : Outport  Port=2
  iz : Outport  Port=3
  is : Outport  Port=4
  wires:
  im/1 -> Gain/1
  Mux2/1 -> Mux/1
  Gain8/1 -> Mux2/2
  iu/1 -> Mux2/1, Gain8/1
  Gain/1 -> Mux/2
  Mux/1 -> Gain7/1, ixy/1
  ie/1 -> Gain6/1
  Sum4/1 -> is/1
  Gain7/1 -> Sum4/1, iB/1
  Gain6/1 -> iz/1, Sum4/2

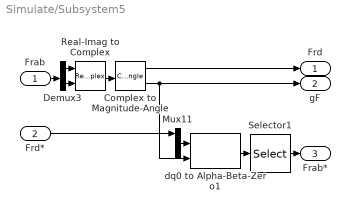
== system Simulate/Subsystem5 ==
  Frab : Inport
  Frd* : Inport  Port=2
  Complex to Magnitude-Angle : ComplexToMagnitudeAngle
  Demux3 : Demux  Outputs=2
  Mux11 : Mux  Inputs=3
  Real-Imag to Complex : RealImagToComplex
  Selector1 : Selector  InputPortWidth=3  IndexOptions=Index vector (dialog)  Indices=[1 2]  OutputSizes=1
  dq0 to Alpha-Beta-Zero1 : spsdq0toAlphaBetaZeroLib/dq0 to Alpha-Beta-Zero  Alignment=90 degrees behind phase A axis
  Frd : Outport
  gF : Outport  Port=2
  Frab* : Outport  Port=3
  wires:
  dq0 to Alpha-Beta-Zero1/1 -> Selector1/1
  Mux11/1 -> dq0 to Alpha-Beta-Zero1/1
  Complex to Magnitude-Angle/2 -> dq0 to Alpha-Beta-Zero1/2, gF/1
  Complex to Magnitude-Angle/1 -> Frd/1
  Selector1/1 -> Frab*/1
  Demux3/2 -> Real-Imag to Complex/2
  Demux3/1 -> Real-Imag to Complex/1
  Real-Imag to Complex/1 -> Complex to Magnitude-Angle/1
  Frab/1 -> Demux3/1
  Frd*/1 -> Mux11/1

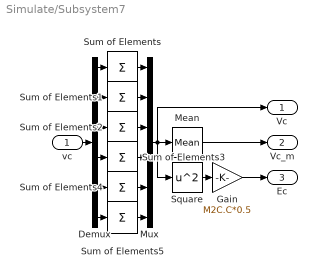
== system Simulate/Subsystem7 ==
  vc : Inport
  Demux : Demux  Outputs=[4; 4; 4; 4; 4; 4]
  Gain : Gain  Gain=M2C.C*0.5
  Mean : dspstat3/Mean  run=off  InputProcessing=Columns as channels (frame based)  reset_popup=None  directionMode=Entire input  dimension=1  roiEnable=off  roiType=Rectangles  roiPortion=Entire ROI  roiOutput=Individual statistics for each ROI  roiFlag=off  roundingMode=Floor  overflowMode=off  outputDataTypeStr=Inherit: Same as accumulator  outputMin=[]  outputMax=[]  outputLastDataTypeStr=Inherit: Same as accumulator
  Mux : Mux  Inputs=6
  Square : Math  Operator=square
  Sum of Elements{,1..5} (6 alike) : Sum  Inputs=+
  Vc : Outport
  Vc_m : Outport  Port=2
  Ec : Outport  Port=3
  wires:
  Square/1 -> Gain/1
  Gain/1 -> Ec/1
  Mean/1 -> Vc_m/1
  vc/1 -> Demux/1
  Demux/1 -> Sum of Elements/1
  Demux/2 -> Sum of Elements1/1
  Demux/3 -> Sum of Elements2/1
  Demux/4 -> Sum of Elements3/1
  Demux/5 -> Sum of Elements4/1
  Demux/6 -> Sum of Elements5/1
  Sum of Elements/1 -> Mux/1
  Sum of Elements1/1 -> Mux/2
  Sum of Elements2/1 -> Mux/3
  Sum of Elements3/1 -> Mux/4
  Sum of Elements4/1 -> Mux/5
  Sum of Elements5/1 -> Mux/6
  Mux/1 -> Vc/1, Square/1, Mean/1

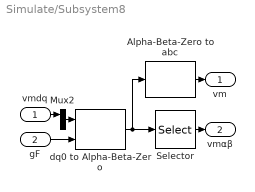
== system Simulate/Subsystem8 ==
  vmdq : Inport
  gF : Inport  Port=2
  Alpha-Beta-Zero to abc : spsAlphaBetaZerotoabcLib/Alpha-Beta-Zero to abc
  Mux2 : Mux  Inputs=[2; 1]
  Selector : Selector  InputPortWidth=3  IndexOptions=Index vector (dialog)  Indices=[1 2]  OutputSizes=1
  dq0 to Alpha-Beta-Zero : spsdq0toAlphaBetaZeroLib/dq0 to Alpha-Beta-Zero  Alignment=Aligned with phase A axis
  vm : Outport
  vmαβ : Outport  Port=2
  wires:
  Mux2/1 -> dq0 to Alpha-Beta-Zero/1
  vmdq/1 -> Mux2/1
  gF/1 -> dq0 to Alpha-Beta-Zero/2
  dq0 to Alpha-Beta-Zero/1 -> Selector/1, Alpha-Beta-Zero to abc/1
  Selector/1 -> vmαβ/1
  Alpha-Beta-Zero to abc/1 -> vm/1

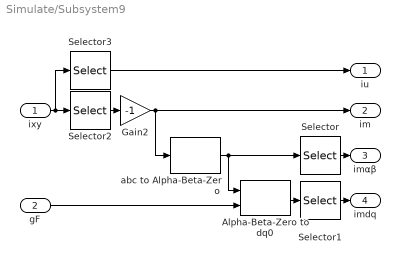
== system Simulate/Subsystem9 ==
  ixy : Inport
  gF : Inport  Port=2
  Alpha-Beta-Zero to dq0 : spsAlphaBetaZerotodq0Lib/Alpha-Beta-Zero to dq0  Alignment=Aligned with phase A axis
  Gain2 : Gain  Gain=-1
  Selector : Selector  InputPortWidth=3  IndexOptions=Index vector (dialog)  Indices=[1 2]  OutputSizes=1
  Selector1 : Selector  InputPortWidth=3  IndexOptions=Index vector (dialog)  Indices=[1 2]  OutputSizes=1
  Selector2 : Selector  InputPortWidth=5  IndexOptions=Index vector (dialog)  Indices=[3 4 5]  OutputSizes=1
  Selector3 : Selector  InputPortWidth=5  IndexOptions=Index vector (dialog)  Indices=[1]  OutputSizes=1
  abc to Alpha-Beta-Zero : spsabctoAlphaBetaZeroLib/abc to Alpha-Beta-Zero
  iu : Outport
  im : Outport  Port=2
  imαβ : Outport  Port=3
  imdq : Outport  Port=4
  wires:
  Selector/1 -> imαβ/1
  Alpha-Beta-Zero to dq0/1 -> Selector1/1
  abc to Alpha-Beta-Zero/1 -> Alpha-Beta-Zero to dq0/1, Selector/1
  gF/1 -> Alpha-Beta-Zero to dq0/2
  ixy/1 -> Selector3/1, Selector2/1
  Selector1/1 -> imdq/1
  Gain2/1 -> im/1, abc to Alpha-Beta-Zero/1
  Selector2/1 -> Gain2/1
  Selector3/1 -> iu/1

== system Simulate/M2C+IM/ CircuitID11  ==

== matlab function Simulate/Modulation index ==
  data: D output; vs input; Vc input; vc input; is input; M2C parameter
function D = delta(vs, Vc, vc, is, M2C)
%#codegen

persistent vc_m_ref m
if isempty(vc_m_ref)
    m = M2C.m;
    Nsm = M2C.Nsm;
    vc_m_ref = M2C.Vc_m_ref / Nsm;
end

vs(4:6) = -vs(4:6);

% Cluster modulation index
D_cluster = min(max(vs ./ Vc, 0), 1);

% Submodule modulation index
D_submodule = repmat(D_cluster', 4, 1);

% vc = reshape(vc, 4, 6);
% M = sort(vc / vc_m_ref, 1, 'descend');
% % M = sort(vc ./ (ones(4, 1)*(Vc'/Nsm)), 1, 'descend');
% D_submodule = zeros(4, 6);
% for k = 1:m
%     if is(k) > 0
%         [~, idxs] = sort(vc(:, k), 'ascend');
%     else
%         [~, idxs] = sort(vc(:, k), 'descend');
%     end
%     D_submodule(:, k) = D_cluster(k) * M(idxs, k);
% end

D = zeros(24, 1);
D(:) = D_submodule(:);
end

== matlab function Simulate/Stator Voltage ==
  data: vm_dq output; imdq_ref input; Frd input; ws input; wm input; IM_vs parameter
function vm_dq = IM_get_vm(imdq_ref, Frd, ws, wm, IM_vs)
%#codegen

M       = IM_vs.M;
M(1, 2) = M(1, 2) * ws;
M(2, 1) = M(2, 1) * ws;
M(2, 3) = M(2, 3) * wm;

vm_dq = M * [imdq_ref;
             Frd];

== matlab function Simulate/Current control Coupled Converter and Motor ==
  data: is_ref input; vo_ref input; vs_ref input; is input; vs output; Vc input; vBx input; Fr_ab input; wm input; flag output; J output; Nac output; Tex output; M2C parameter; CCMPC parameter; IM parameter; RFT parameter
function [vs, flag, J, Nac, Tex] = CMPC(is_ref, vo_ref, vs_ref, is, Vc, vBx, Fr_ab, wm, M2C, CCMPC, IM, RFT)
%#codegen

% CMPC: Cluster Current Model Predictive Control

% vs:   control action
% flag: solver verbose
% J:    cost function
% Nac:  # of active constraints
% Tex:  Execution time

% Initialization

persistent Ad Bd is_max Vc_m_ref lambda m Hx Hu H Aineq iA options Mv Mf np
if isempty(Ad)
    Ad       = CCMPC.Ad;                  % Discrete state matrix
    Bd       = CCMPC.Bd;                  % Discrete input matrix
    is_max   = M2C.is_max;                % Max. cluster current
    Vc_m_ref = M2C.Vc_m_ref;              % Max. cluster capacitor voltage
    lambda   = CCMPC.lambda;              % Control effort weighting factor
    m        = M2C.m;                     % # of converter clusters
    Hx       = CCMPC.Hx;                  % Reference tracking hessian
    Hu       = CCMPC.Hu;                  % Control effort hessian
    H        = CCMPC.H;                   % Total hessian
    Aineq    = CCMPC.Aineq;               % Control actions constraints matrix
    iA       = false(size(Aineq, 1), 1);  % Active constraints
    options  = mpcActiveSetOptions;       % mpcActiveSetSolver options
    options.MaxIterations       = 100;
    options.ConstraintTolerance = 1.0e-5;
    Mv       = -IM.kr * M2C.ay' * RFT.ab2abc;
    Mf       = 1/IM.tau_r * eye(2);
    np       = IM.np;
end

tic

we       = wm * np;
Mf(1, 2) = we;
Mf(2, 1) = -we;
vBy      = Mv * Mf * Fr_ab;
vB       = vBx - vBy;

% Reference tracking linear term, normalized
fx = 2 * Bd' * (-is_ref + Ad * is - Bd * vB) / is_max^2;

% Control effort linear term, normalized
fu = -2 * vs_ref / Vc_m_ref^2;

% Total weighted linear term
f = fx + lambda * fu;

% Control action constraints
ub    = [Vc(1:3); 0; 0; 0] + vo_ref;
lb    = [0; 0; 0; -Vc(4:6)] + vo_ref;
bineq = [ub; -lb];

% Solve
[vsp, flag, iA, ~] = mpcActiveSetSolver(H, f, Aineq, bineq, zeros(0, m), zeros(0, 1), iA, options);
vs = vsp - vo_ref;

% Control summary
Tex = toc;
Nac = sum(iA);
Jx = vsp' * Hx * vsp + fx' * vsp;
Ju = vsp' * Hu * vsp + fu' * vsp;
J  =  Jx + lambda * Ju;
end

== matlab function Simulate/Subsystem1/MATLAB Function ==
  data: iB_ref input; iz_max output; M2C parameter; iz_min output
function [iz_max, iz_min] = iz_lim(iB_ref, M2C)
%#codegen

persistent is_max
if isempty(is_max)
    is_max = M2C.is_max;
end

iz_max = is_max - iB_ref;
iz_min = -is_max - iB_ref;

== matlab function Simulate/Current control Decoupled model ==
  data: iu_ref input; imab_ref input; ie_ref input; iu input; vs output; im_ab input; ie input; Fr_ab input; wm input; Vdc input; vo_ref input; vs_ref input; Vc input; CCMPC parameter; M2C parameter; flag output; J output; Nac output; Tex output
function [vs, flag, J, Nac, Tex] = CMPC(iu_ref, imab_ref, ie_ref, iu, im_ab, ie, Fr_ab, wm, Vdc, vo_ref, vs_ref, Vc, CCMPC, M2C)
%#codegen

persistent m Ad Bd integrated H Hx Hu is_max Aineq iA options Vc_m_ref lambda Wx
if isempty(m)
    m = M2C.m;
    Ad = CCMPC.Ad;
    Bd = CCMPC.Bd;
    integrated = CCMPC.integrated;
    H = CCMPC.H;
    Wx = CCMPC.Wx;
    Hx = CCMPC.Hx;
    Hu = CCMPC.Hu;
    is_max = M2C.is_max;
    Vc_m_ref = M2C.Vc_m_ref;              % Max. cluster capacitor voltage
    lambda   = CCMPC.lambda;              % Control effort weighting factor
    Aineq    = CCMPC.Aineq;               % Control actions constraints matrix
    iA       = false(size(Aineq, 1), 1);  % Active constraints
    options  = mpcActiveSetOptions;       % mpcActiveSetSolver options
    options.MaxIterations       = 100;
    options.ConstraintTolerance = 1.0e-5;
end

tic

Es = CCMPC.Es;
Es(2, 3) = Es(2, 3)*wm;
Es(3, 2) = Es(3, 2)*wm;
Ed = integrated*Es;

x_ref = [iu_ref;
         imab_ref;
         ie_ref];

x = [iu;
     im_ab;
     ie];

p = [Vdc;
     Fr_ab];

% Reference tracking linear term, normalized
fx = 2 * Bd' * Wx * (-x_ref + Ad * x + Ed * p) / is_max^2;

% Control effort linear term, normalized
fu = -2 * vs_ref / Vc_m_ref^2;

% Total weighted linear term
f = fx + lambda * fu;

% Control action constraints
% ub    = [Vc(1:3); 0; 0; 0] + vo_ref;
% lb    = [0; 0; 0; -Vc(4:6)] + vo_ref;
ub    = [Vc(1:3); 0; 0; 0] - vo_ref;
lb    = [0; 0; 0; -Vc(4:6)] - vo_ref;
bineq = [ub; -lb];

% Solve
[vsp, flag, iA, ~] = mpcActiveSetSolver(H, f, Aineq, bineq, zeros(0, m), zeros(0, 1), iA, options);
% vs = vsp - vo_ref;
vs = vsp + vo_ref;

% Control summary
Tex = toc;
Nac = sum(iA);
Jx = vsp' * Hx * vsp + fx' * vsp;
Ju = vsp' * Hu * vsp + fu' * vsp;
J  =  Jx + lambda * Ju;
end

== matlab function Simulate/Subsystem2/MATLAB Function ==
  data: Vc input; vs_max output; vo_ref input; vs_min output
function [vs_max, vs_min] = vs_lim(Vc, vo_ref)

vs_max = [Vc(1:3); zeros(3, 1)] + vo_ref;
vs_min = [zeros(3, 1); -Vc(4:6)] + vo_ref;
